simulink model "test_frictionmodel"  (R2018b)
settings: configuration reference "Physics" (kept outside this file)
model workspace (MAT data in the model file):
  veh_param = Simulink.Parameter
  veh_param.Value.cLiftF = 0
  veh_param.Value.cLiftR = 0
  veh_param.Value.CoGx_m = 0
  veh_param.Value.CoGy_m = 0
  veh_param.Value.CoGz_m = 0
  veh_param.Value.cDrag = 0
  veh_param.Value.Aref_m2 = 0
  veh_param.Value.Gearratio = 0
  veh_param.Value.Wheelbase_m = 0
  veh_param.Value.PacLatF = [0 0 0 0 0]
  veh_param.Value.PacLongF = [0 0 0 0 0]
  veh_param.Value.PacLatR = [0 0 0 0 0]
  veh_param.Value.PacLongR = [0 0 0 0 0]
  veh_param.Value.cRollFriction_Npmps = 0
  veh_param.Value.MaxRollFriction_N = 0
  veh_param.Value.T_YawRate_s = 0
  veh_param.Value.T_LatVel_s = 0
  veh_param.Value.TrackWidthF_m = 0
  veh_param.Value.TrackWidthR_m = 0
  veh_param.Value.TireRadiusF_m = 0
  veh_param.Value.TireRadiusR_m = 0
  veh_param.Value.VehicleInertia_kgm2 = 0
  veh_param.Value.WheelInertiaF_kgm2 = 0
  veh_param.Value.WheelInertiaR_kgm2 = 0
  veh_param.Value.VehicleMass_kg = 0
  veh_param.Value.switchModelBlend_mps = 0
  veh_param.Value.PTLimitLowVel_N = 0
  veh_param.Value.switchModelVel_mps = 0
  veh_param.Value.T_Tire_s = 0
  veh_param.DataType = 'struct'
  veh_param.Dimensions = [1 1]
  x0_positionstates = Simulink.Parameter
  x0_positionstates.Value = [0 0 0]
  x0_positionstates.DataType = 'auto'
  x0_positionstates.Dimensions = [1 3]
settings Model: DataDictionary=test_frictionmodel.sldd  OrderedModelArguments=off  Creator=wischnewski  LastModifiedBy=staer

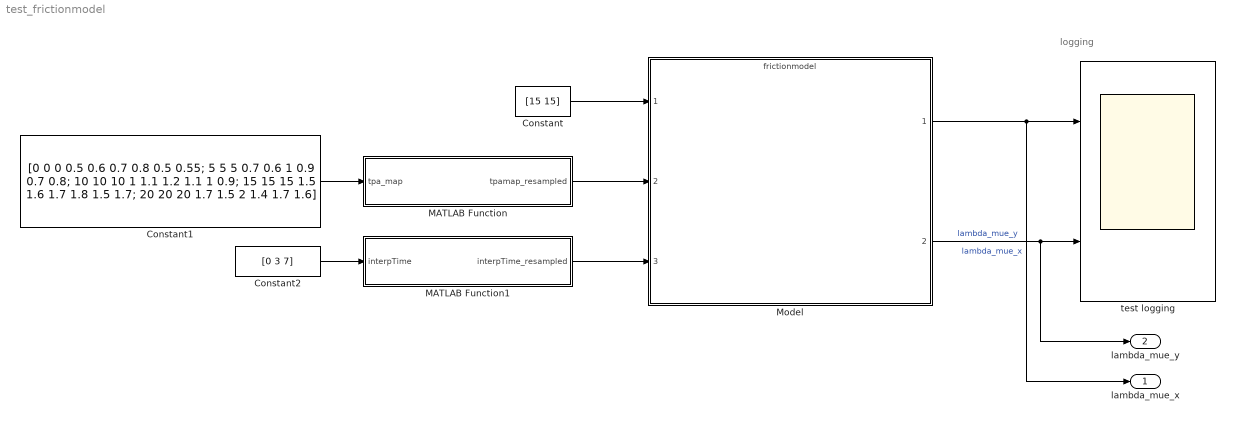
== system test_frictionmodel ==
  note: logging
  Constant : Constant  Value=[15 15]
  Constant1 : Constant  Value=[0 0 0 0.5 0.6 0.7 0.8 0.5 0.55; 5 5 5 0.7 0.6 1 0.9 0.7 0.8; 10 10 10 1 1.1 1.2 1.1 1 0.9; 15 15 15 1.5 1.6 1.7 1.8 1.5 1.7; 20 20 20 1.7 1.5 2 1.4 1.7 1.6]
  Constant2 : Constant  Value=[0 3 7]
  MATLAB Function : MATLAB Function  TreatAsAtomicUnit=on
  MATLAB Function1 : MATLAB Function  TreatAsAtomicUnit=on
  Model : ModelReference  ModelNameDialog=frictionmodel  SimulationMode=Normal  ModelReferenceVersion=1.389
  test logging : Scope  NumInputPorts=2
  lambda_mue_x : Outport
  lambda_mue_y : Outport  Port=2
  wires:
  Constant/1 -> Model/1
  Model/1 -> lambda_mue_x/1, test logging/1  "lambda_mue_x"
  Model/2 -> lambda_mue_y/1, test logging/2  "lambda_mue_y"
  Constant1/1 -> MATLAB Function/1(tpa_map)
  Constant2/1 -> MATLAB Function1/1(interpTime)
  MATLAB Function/1(tpamap_resampled) -> Model/2
  MATLAB Function1/1(interpTime_resampled) -> Model/3

== matlab function test_frictionmodel/MATLAB Function1 ==
  data: interpTime input; interpTime_resampled output
function interpTime_resampled = fcn(interpTime)

interpTime_resampled    = zeros(1,10);
tpamap_size             = length(interpTime);
interpTime_resampled(1:tpamap_size) = ...
    interpTime(1:tpamap_size);

== matlab function test_frictionmodel/MATLAB Function ==
  data: tpa_map input; tpamap_resampled output
function tpamap_resampled = fcn(tpa_map)

tpamap_resampled    = zeros(2500,23);
tpamap_size         = size(tpa_map);
tpamap_resampled(1:tpamap_size(1),1:tpamap_size(2)) = ...
    tpa_map(1:tpamap_size(1),1:tpamap_size(2));
